simulink model "MAS1"  (R2021b)
settings: Solver=VariableStepAuto  StartTime=0.0  StopTime=15  RelTol=1e-3
libraries: cstblocks x3
settings Model: Creator=lenovo  LastModifiedBy=lenovo

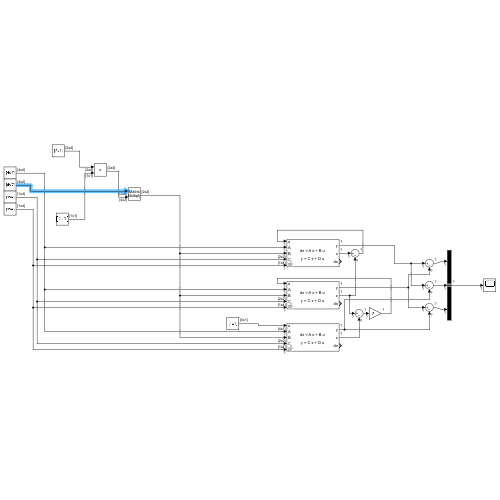
[thumbnail: Simulink's stored preview of the top-level diagram]
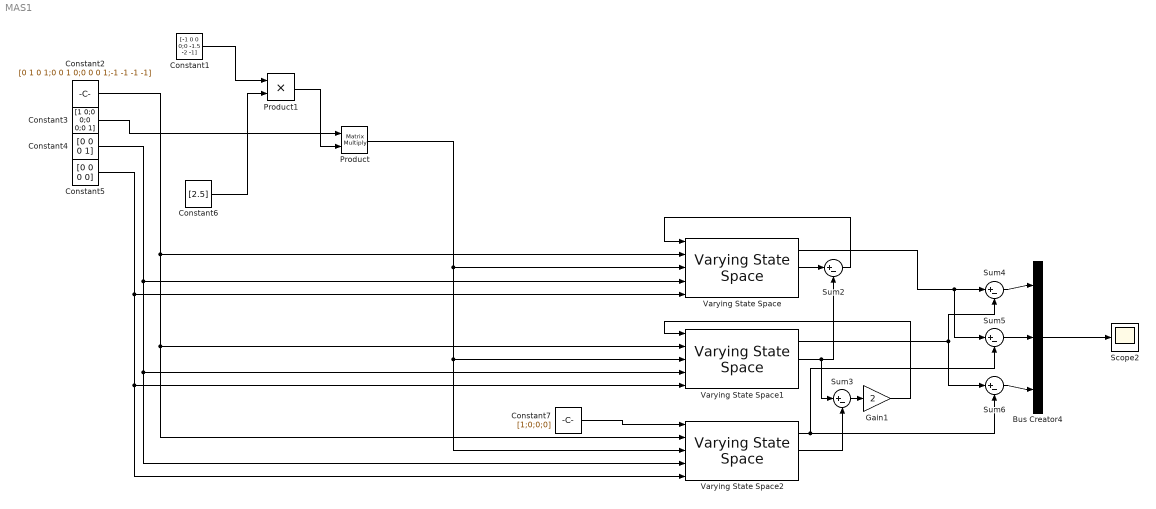
== system MAS1 ==
  Bus Creator4 : BusCreator  Inputs=3
  Constant1 : Constant  Value=[-1 0 0 0;0 -1.5 -2 -1]
  Constant2 : Constant  Value=[0 1 0 1;0 0 1 0;0 0 0 1;-1 -1 -1 -1]
  Constant3 : Constant  Value=[1 0;0 0;0 0;0 1]
  Constant4 : Constant  Value=[0 0 0 1]  VectorParams1D=off
  Constant5 : Constant  Value=[0 0 0 0]  VectorParams1D=off
  Constant6 : Constant  Value=[2.5]  VectorParams1D=off
  Constant7 : Constant  Value=[1;0;0;0]  VectorParams1D=off
  Gain1 : Gain  Gain=2
  Product : Product  Multiplication=Matrix(*)
  Product1 : Product
  Scope2 : Scope
  Sum{2..6} (5 alike) : Sum  Inputs=|+-
  Varying State Space : cstblocks/Linear Parameter Varying/Varying State Space  x0=0  xNames=''  OutputX=on  OutputDX=on
  Varying State Space1 : cstblocks/Linear Parameter Varying/Varying State Space  x0=0  xNames=''  OutputX=on  OutputDX=on
  Varying State Space2 : cstblocks/Linear Parameter Varying/Varying State Space  x0=0  xNames=''  OutputX=on  OutputDX=on
  wires:
  Constant2/1 -> Varying State Space2/2, Varying State Space1/2, Varying State Space/2
  Constant4/1 -> Varying State Space2/4, Varying State Space1/4, Varying State Space/4
  Constant5/1 -> Varying State Space2/5, Varying State Space1/5, Varying State Space/5
  Constant7/1 -> Varying State Space2/1
  Bus Creator4/1 -> Scope2/1
  Varying State Space1/2 -> Sum2/2, Sum3/1
  Sum2/1 -> Varying State Space/1
  Sum3/1 -> Gain1/1
  Gain1/1 -> Varying State Space1/1
  Constant3/1 -> Product/1
  Constant6/1 -> Product1/2
  Product/1 -> Varying State Space2/3, Varying State Space1/3, Varying State Space/3
  Varying State Space2/2 -> Sum3/2
  Varying State Space/2 -> Sum2/1
  Varying State Space/1 -> Sum5/1, Sum4/1
  Varying State Space1/1 -> Sum6/1, Sum4/2
  Varying State Space2/1 -> Sum6/2, Sum5/2
  Sum4/1 -> Bus Creator4/1
  Sum5/1 -> Bus Creator4/2
  Sum6/1 -> Bus Creator4/3
  Constant1/1 -> Product1/1
  Product1/1 -> Product/2
